simulink model "control_observador"  (R2022a)
settings: Solver=VariableStepAuto  StartTime=0.0  StopTime=1.5  RelTol=1e-3
values from neighbouring files (symbols this model uses):
  A = sys.A    [RealEstadoObserServoTipo0.m]
  B = sys.B    [RealEstadoObserServoTipo0.m]
  C = sys.C    [RealEstadoObserServoTipo0.m]    (also in control 2 tf.mat = 0.0033)
  Ke = acker(A',C',[-30 -30 -30])'    [RealEstadoObserServoTipo0.m]
  Ki = -Khat(m)    [RealEstadoObserServoTipo0.m]
undefined symbols (not defined in the file or in its folder): Kc
settings Model: Creator=Juan Andres  LastModifiedBy=niorc
settings SolverCC: AlgebraicLoopSolver=TrustRegion
settings DebuggingCC: UnconnectedInputMsg=warning  UnconnectedOutputMsg=warning  UnconnectedLineMsg=warning  SFMachineParentedDataDiag=warning

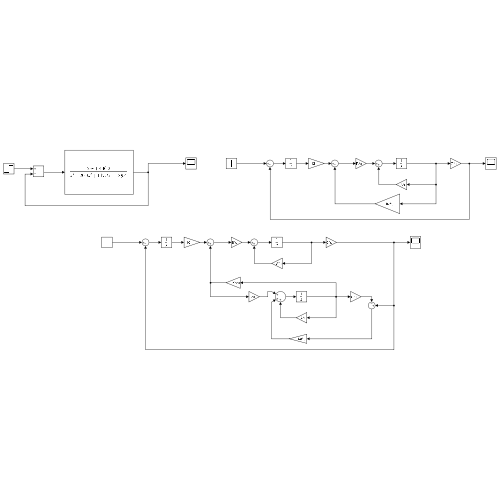
[thumbnail: Simulink's stored preview of the top-level diagram]
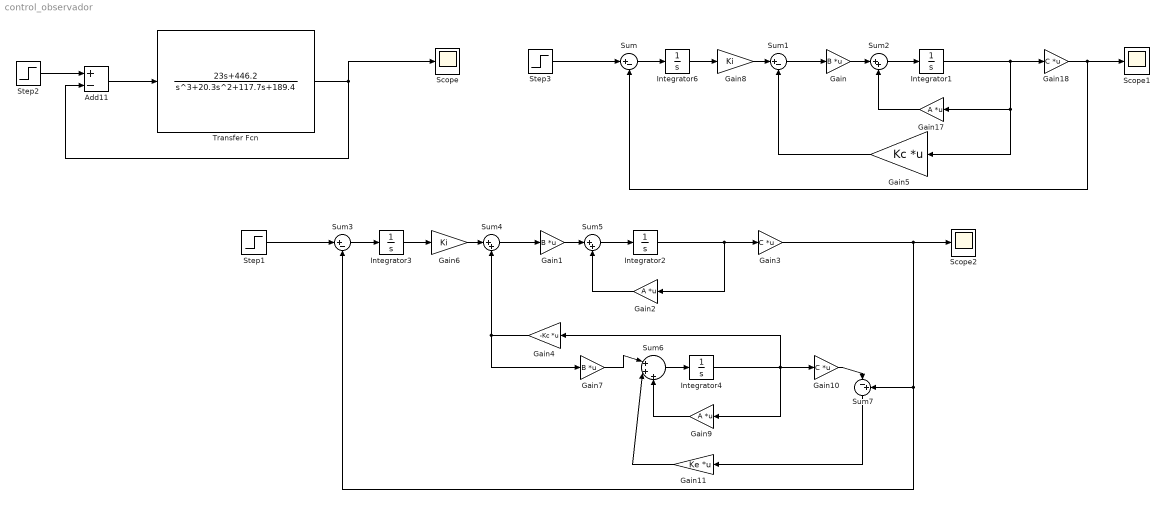
== system control_observador ==
  Add11 : Sum  Inputs=+-
  Gain : Gain  Gain=B  Multiplication=Matrix(K*u)
  Gain1 : Gain  Gain=B  Multiplication=Matrix(K*u)
  Gain10 : Gain  Gain=C  Multiplication=Matrix(K*u)
  Gain11 : Gain  Gain=Ke  Multiplication=Matrix(K*u)
  Gain17 : Gain  Gain=A  Multiplication=Matrix(K*u)
  Gain18 : Gain  Gain=C  Multiplication=Matrix(K*u)
  Gain2 : Gain  Gain=A  Multiplication=Matrix(K*u)
  Gain3 : Gain  Gain=C  Multiplication=Matrix(K*u)
  Gain4 : Gain  Gain=-Kc  Multiplication=Matrix(K*u)
  Gain5 : Gain  Gain=Kc  Multiplication=Matrix(K*u)
  Gain6 : Gain  Gain=Ki
  Gain7 : Gain  Gain=B  Multiplication=Matrix(K*u)
  Gain8 : Gain  Gain=Ki
  Gain9 : Gain  Gain=A  Multiplication=Matrix(K*u)
  Integrator1 : Integrator  InitialCondition=[0;0;0]
  Integrator2 : Integrator  InitialCondition=[0;0;0]
  Integrator3 : Integrator
  Integrator4 : Integrator  InitialCondition=[0;0;0]
  Integrator6 : Integrator
  Scope : Scope
  Scope1 : Scope
  Scope2 : Scope
  Step1 : Step  Time=0  SampleTime=0
  Step2 : Step  Time=0  SampleTime=0
  Step3 : Step  Time=0  SampleTime=0
  Sum : Sum  Inputs=|+-
  Sum1 : Sum  Inputs=|+-
  Sum2 : Sum  Inputs=|++
  Sum3 : Sum  Inputs=|+-
  Sum4 : Sum  Inputs=|++
  Sum5 : Sum  Inputs=|++
  Sum6 : Sum  Inputs=|+++
  Sum7 : Sum  Inputs=|-+
  Transfer Fcn : TransferFcn  Numerator=[23 446.2]  Denominator=[1 20.3 117.7 189.4]
  wires:
  Step2/1 -> Add11/1
  Add11/1 -> Transfer Fcn/1
  Transfer Fcn/1 -> Add11/2, Scope/1
  Gain18/1 -> Scope1/1, Sum/2
  Integrator6/1 -> Gain8/1
  Sum2/1 -> Integrator1/1
  Integrator1/1 -> Gain5/1, Gain17/1, Gain18/1
  Sum/1 -> Integrator6/1
  Step3/1 -> Sum/1
  Gain5/1 -> Sum1/2
  Gain8/1 -> Sum1/1
  Sum1/1 -> Gain/1
  Gain17/1 -> Sum2/2
  Gain/1 -> Sum2/1
  Sum3/1 -> Integrator3/1
  Step1/1 -> Sum3/1
  Gain6/1 -> Sum4/1
  Sum5/1 -> Integrator2/1
  Gain1/1 -> Sum5/1
  Gain2/1 -> Sum5/2
  Sum4/1 -> Gain1/1
  Integrator2/1 -> Gain2/1, Gain3/1
  Integrator3/1 -> Gain6/1
  Gain3/1 -> Scope2/1, Sum7/2, Sum3/2
  Integrator4/1 -> Gain4/1, Gain9/1, Gain10/1
  Gain4/1 -> Gain7/1, Sum4/2
  Sum6/1 -> Integrator4/1
  Gain7/1 -> Sum6/1
  Gain10/1 -> Sum7/1
  Sum7/1 -> Gain11/1
  Gain9/1 -> Sum6/3
  Gain11/1 -> Sum6/2
